simulink model "kuangtu"  (R2015b)
settings: Solver=VariableStepAuto  StartTime=0.0  StopTime=10.0  RelTol=1e-3
undefined symbols (not defined in the file or in its folder): Gc, H1, H2, J, K2, Kc, Kt, s
settings Model: Creator=朱明菲  LastModifiedBy=29118

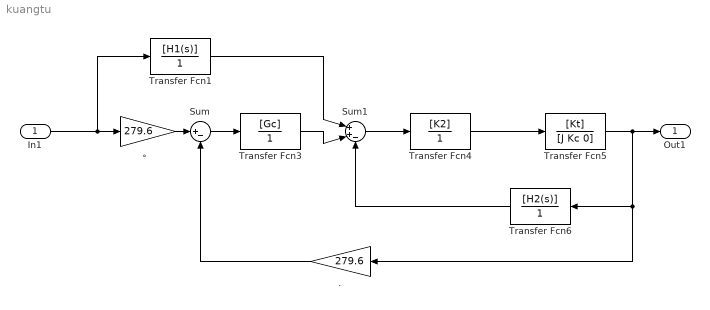
== system kuangtu ==
  In1 : Inport
  ". " : Gain  Gain=279.6
  Sum : Sum  Inputs=|+-
  Sum1 : Sum  Inputs=|++-
  Transfer Fcn1 : TransferFcn  Numerator=[H1(s)]  Denominator=[1]
  Transfer Fcn3 : TransferFcn  Numerator=[Gc]  Denominator=[1]
  Transfer Fcn4 : TransferFcn  Numerator=[K2]  Denominator=[1]
  Transfer Fcn5 : TransferFcn  Numerator=[Kt]  Denominator=[J Kc 0]
  Transfer Fcn6 : TransferFcn  Numerator=[H2(s)]  Denominator=[1]
  。 : Gain  Gain=279.6
  Out1 : Outport
  wires:
  。/1 -> Sum/1
  Sum/1 -> Transfer Fcn3/1
  Sum1/1 -> Transfer Fcn4/1
  Transfer Fcn4/1 -> Transfer Fcn5/1
  In1/1 -> Transfer Fcn1/1, 。/1
  ". "/1 -> Sum/2
  Transfer Fcn5/1 -> Transfer Fcn6/1, ". "/1, Out1/1
  Transfer Fcn1/1 -> Sum1/1
  Transfer Fcn3/1 -> Sum1/2
  Transfer Fcn6/1 -> Sum1/3
